simulink model "Sub1"  (R2024a)
settings: Solver=FixedStepDiscrete  StartTime=0.0  StopTime=1  FixedStep=7.5e-05  RelTol=1e-3  EnableMultiTasking=on
undefined symbols (not defined in the file or in its folder): D1, D11, Delta
libraries: spsSeriesRLCBranchLib x41, spsLoadFlowBusLib x29, spsDistributedParametersLineLib x19, spsThreePhaseSeriesRLCLoadLib x15, spsThreePhaseTransformerTwoWindingsLib x13, spsThreePhaseParallelRLCLoadLib x11, spsThreePhaseVIMeasurementLib x11, spsSynchronousMachinepuStandardLib x7, spsExcitationSystemLib x7, spsHydraulicTurbineandGovernorLib x7, spsGenericPowerSystemStabilizerLib x7, spsMultiBandPowerSystemStabilizerLib x7
(part 2 of 5)

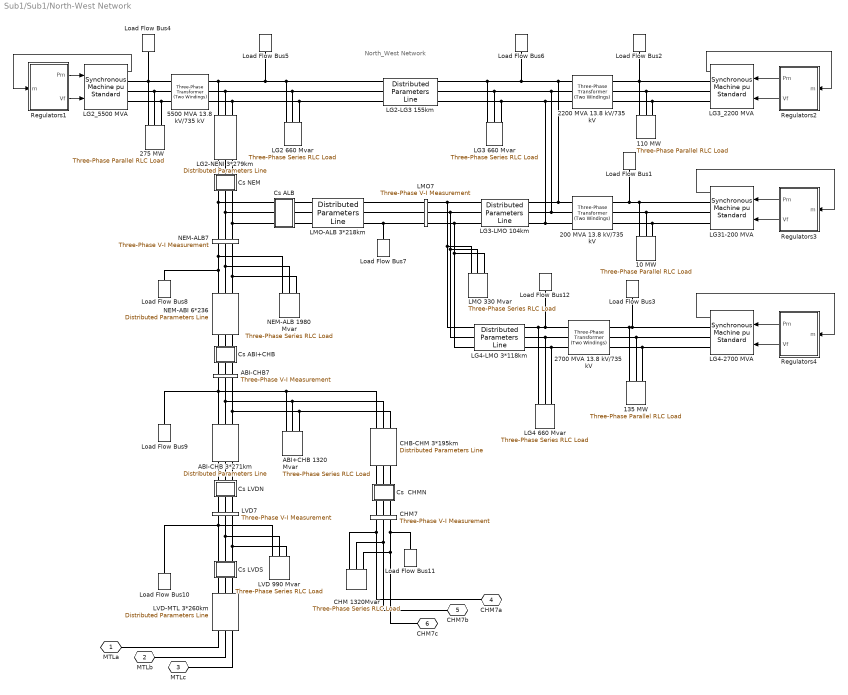
== system Sub1/Sub1/North-West Network ==
  note: North_West Network
  10 MW : spsThreePhaseParallelRLCLoadLib/Three-Phase Parallel RLC Load  LConnTagsString=A|B|C  Configuration=Y (grounded)  NominalVoltage=(13800)*1  Vabc=[1e3 1e3 1e3]  Vabcp=[1e3 1e3 1e3]  NominalFrequency=60  UnbalancedPower=off  ActivePower=10000000  InductivePower=0  CapacitivePower=0  Pabc=[10e3 9e3 11e3]  QLabc=[100 90 110]  QCabc=[100 90 110]  Pabcp=[10e3 9e3 11e3]  QLabcp=[100 90 110]  QCabcp=[100 90 110]  Measurements=None  LoadType=constant PQ
  110 MW : spsThreePhaseParallelRLCLoadLib/Three-Phase Parallel RLC Load  LConnTagsString=A|B|C  Configuration=Y (grounded)  NominalVoltage=(13800)*1  Vabc=[1e3 1e3 1e3]  Vabcp=[1e3 1e3 1e3]  NominalFrequency=60  UnbalancedPower=off  ActivePower=110000000  InductivePower=0  CapacitivePower=0  Pabc=[10e3 9e3 11e3]  QLabc=[100 90 110]  QCabc=[100 90 110]  Pabcp=[10e3 9e3 11e3]  QLabcp=[100 90 110]  QCabcp=[100 90 110]  Measurements=None  LoadType=constant PQ
  135 MW : spsThreePhaseParallelRLCLoadLib/Three-Phase Parallel RLC Load  LConnTagsString=A|B|C  Configuration=Y (grounded)  NominalVoltage=(13800)*1  Vabc=[1e3 1e3 1e3]  Vabcp=[1e3 1e3 1e3]  NominalFrequency=60  UnbalancedPower=off  ActivePower=135000000  InductivePower=0  CapacitivePower=0  Pabc=[10e3 9e3 11e3]  QLabc=[100 90 110]  QCabc=[100 90 110]  Pabcp=[10e3 9e3 11e3]  QLabcp=[100 90 110]  QCabcp=[100 90 110]  Measurements=None  LoadType=constant PQ
  200 MVA 13.8 kV/735 kV : spsThreePhaseTransformerTwoWindingsLib/Three-Phase Transformer (Two Windings)  Winding1Connection=Delta (D1)  Winding2Connection=Yg  CoreType=Three single-phase transformers  SetSaturation=off  Hysteresis=off  DataFile='basic_model'  SetInitialFlux=off  Measurements=None  UNITS=pu  NominalPower=[ 200e6 60 ]  Winding1="[ 13.8e3 0.002  0.0]"  Winding2=[ 735e3 0.002 0.12]  Rm=500  Lm=500  L0=0.5  Saturation="[ 0,0  ;  0.005,1.2  ;  1.0,1.4 ]"  InitialFluxes=[ 0.8 , -0.8 , 0.7 ]  BreakLoop=off  DiscreteSolver=Trapezoidal iterative  DataType=off  TransfoNumber=0
  2200 MVA 13.8 kV/735 kV : spsThreePhaseTransformerTwoWindingsLib/Three-Phase Transformer (Two Windings)  Winding1Connection=Delta (D1)  Winding2Connection=Yg  CoreType=Three single-phase transformers  SetSaturation=off  Hysteresis=off  DataFile='basic_model'  SetInitialFlux=off  Measurements=None  UNITS=pu  NominalPower=[ 2200e6 60 ]  Winding1="[ 13.8e3 0.002  0.0]"  Winding2=[ 735e3 0.002 0.12]  Rm=500  Lm=500  L0=0.5  Saturation="[ 0,0  ;  0.005,1.2  ;  1.0,1.4 ]"  InitialFluxes=[ 0.8 , -0.8 , 0.7 ]  BreakLoop=off  DiscreteSolver=Trapezoidal iterative  DataType=off  TransfoNumber=0
  2700 MVA 13.8 kV/735 kV : spsThreePhaseTransformerTwoWindingsLib/Three-Phase Transformer (Two Windings)  Winding1Connection=Delta (D1)  Winding2Connection=Yg  CoreType=Three single-phase transformers  SetSaturation=off  Hysteresis=off  DataFile='basic_model'  SetInitialFlux=off  Measurements=None  UNITS=pu  NominalPower=[ 2700e6 60 ]  Winding1="[ 13.8e3 0.002  0.0]"  Winding2=[ 735e3 0.002 0.12]  Rm=500  Lm=500  L0=0.5  Saturation="[ 0,0  ;  0.005,1.2  ;  1.0,1.4 ]"  InitialFluxes=[ 0.8 , -0.8 , 0.7 ]  BreakLoop=off  DiscreteSolver=Trapezoidal iterative  DataType=off  TransfoNumber=0
  275 MW : spsThreePhaseParallelRLCLoadLib/Three-Phase Parallel RLC Load  LConnTagsString=A|B|C  Configuration=Y (grounded)  NominalVoltage=(13800)*1  Vabc=[1e3 1e3 1e3]  Vabcp=[1e3 1e3 1e3]  NominalFrequency=60  UnbalancedPower=off  ActivePower=275000000  InductivePower=0  CapacitivePower=0  Pabc=[10e3 9e3 11e3]  QLabc=[100 90 110]  QCabc=[100 90 110]  Pabcp=[10e3 9e3 11e3]  QLabcp=[100 90 110]  QCabcp=[100 90 110]  Measurements=None  LoadType=constant PQ
  5500 MVA 13.8 kV/735 kV : spsThreePhaseTransformerTwoWindingsLib/Three-Phase Transformer (Two Windings)  Winding1Connection=Delta (D1)  Winding2Connection=Yg  CoreType=Three single-phase transformers  SetSaturation=off  Hysteresis=off  DataFile='basic_model'  SetInitialFlux=off  Measurements=None  UNITS=pu  NominalPower=[ 5500e6 60 ]  Winding1="[ 13.8e3 0.002  0.0]"  Winding2=[ 735e3 0.002 0.12]  Rm=500  Lm=500  L0=0.5  Saturation="[ 0,0  ;  0.005,1.2  ;  1.0,1.4 ]"  InitialFluxes=[ 0.8 , -0.8 , 0.7 ]  BreakLoop=off  DiscreteSolver=Trapezoidal iterative  DataType=off  TransfoNumber=0
  ABI+CHB 1320 Mvar : spsThreePhaseSeriesRLCLoadLib/Three-Phase Series RLC Load  LConnTagsString=A|B|C  Configuration=Y (grounded)  NominalVoltage=735e3  Vabc=[1e3 1e3 1e3]  Vabcp=[1e3 1e3 1e3]  NominalFrequency=60  UnbalancedPower=off  ActivePower=4400000  InductivePower=1320e6  CapacitivePower=0  Pabc=[10e3 9e3 11e3]  QLabc=[100 90 110]  QCabc=[100 90 110]  Pabcp=[10e3 9e3 11e3]  QLabcp=[100 90 110]  QCabcp=[100 90 110]  Measurements=None  LoadType=constant Z
  ABI-CHB 3*271km : spsDistributedParametersLineLib/Distributed Parameters Line  Phases=3  Length=271  Frequency=60  Resistance="[0.01273  0.3864]/3"  Inductance="[0.9337e-3  4.1264e-3]/3"  Capacitance=[12.74e-9 7.751e-9]*3  x1=[-0.001575 2.7348412269526e-08 -34814.2579741144 -747194.944177871;-0.0015 2.74950573148694e-08 -13676.7298714156 -747880.497252537;-0.001425 2.76197232320838e-08 7471.73119988141 -747968.206100654;-0.00135 2.77223103651424e-08 28614.2194835787 -747458.000609112;-0.001275 2.78027367074606e-08 49733.8339980329 -746350.288628374;-0.0012 2.78609379674511e-08 70813.6920465424 -744645.955646449;-0.001125 2.7896867619917e-08 91836.9427131156 -742346.364081045;-0.00105 2.7910496943244e-08 112786.780332836 -739453.352190476;-0.000975 2.79018150423594e-08 133646.457926055 -735969.23260418;-0.0009 2.78708288574421e-08 154399.300585666 -731896.790474048;-0.000825 2.78175631583741e-08 175028.718806778 -727239.281248007;-0.00075 2.77420605249403e-08 195518.221748105 -722000.428067671;-0.000675 2.76443813127906e-08 215851.430414496 -716184.418792115;-0.0006 2.75246036051927e-08 236012.09075005 -709795.902650165;-0.000525 2.73828231506133e-08 255984.086631366 -702839.986523878;-0.00045 2.72191532861786e-08 275751.452750516 -695322.230866176;-0.000375 2.7033724847074e-08 295298.387377476 -687248.645255907;-0.0003 2.68266860619564e-08 314609.264991783 -678625.683593877;-0.000225 2.6598202434463e-08 333668.64877334 -669460.238943703;-0.00015 2.63484566109096e-08 352461.302942368 -659759.638021603;-7.5e-05 2.60776482342864e-08 370972.204938663 -649531.635339529]  x2=[-0.001575 6.20449125576539e-08 -284619.341076147 -691578.758256562;-0.0015 6.22834048516216e-08 -264954.25531134 -699348.683850865;-0.001425 6.2472108744719e-08 -245077.369168772 -706559.560807692;-0.00135 6.26108733899411e-08 -225004.5719271 -713205.624862332;-0.001275 6.26995878609538e-08 -204751.909473316 -719281.56325287;-0.0012 6.27381812407664e-08 -184335.571475907 -724782.518967121;-0.001125 6.27266226784214e-08 -163771.87844309 -729704.094625253;-0.00105 6.26649214136568e-08 -143077.268676438 -734042.355994989;-0.000975 6.25531267695196e-08 -122268.285130363 -737793.835136568;-0.0009 6.23913281129378e-08 -101361.562187922 -740955.533174962;-0.000825 6.21796547832818e-08 -80373.8123635515 -743524.922697137;-0.00075 6.19182759889726e-08 -59321.8129433384 -745499.949772419;-0.000675 6.16074006722193e-08 -38222.3925735125 -746879.035594386;-0.0006 6.12472773419935e-08 -17092.4178078855 -747661.077742931;-0.000525 6.08381938753752e-08 4051.22037501424 -747845.451065526;-0.00045 6.03804772874285e-08 25191.620074332 -747432.008176959;-0.000375 5.98744934697906e-08 46311.8819780071 -746421.079577148;-0.0003 5.93206468981833e-08 67395.1228718245 -744813.473386949;-0.000225 5.8719380309082e-08 88424.489135598 -742610.474702152;-0.00015 5.80711743457983e-08 109383.170215697 -739813.8445662;-7.5e-05 5.73765471742613e-08 130254.412063144 -736425.818562433]  x3=[-0.001575 1.23942804838449e-10 -354.964030660947 -109.750554352367;-0.0015 1.32024870831634e-10 -351.719210477296 -119.741131836523;-0.001425 1.40001398163125e-10 -348.193231338274 -129.63599009199;-0.00135 1.47866010519017e-10 -344.388911857655 -139.427219320474;-0.001275 1.55612421048526e-10 -340.309293150224 -149.106992563141;-0.0012 1.63234437389599e-10 -335.957636400756 -158.667571957367;-0.001125 1.70725966618993e-10 -331.337420257073 -168.101314922266;-0.00105 1.78081020122867e-10 -326.452338049269 -177.400680268052;-0.000975 1.85293718383986e-10 -321.306294837316 -186.558234224353;-0.0009 1.92358295681718e-10 -315.903404289422 -195.566656382652;-0.000825 1.99269104701062e-10 -310.247985393623 -204.418745548109;-0.00075 2.06020621047027e-10 -304.344559005254 -213.107425496086;-0.000675 2.12607447660749e-10 -298.197844233044 -221.625750628775;-0.0006 2.19024319133814e-10 -291.812754666734 -229.966911527399;-0.000525 2.25266105917348e-10 -285.194394449229 -238.12424039556;-0.00045 2.31327818422499e-10 -278.348054196421 -246.091216389371;-0.000375 2.37204611009036e-10 -271.279206767956 -253.861470830122;-0.0003 2.42891785858886e-10 -263.993502892313 -261.428792295303;-0.000225 2.48384796731489e-10 -256.496766649693 -268.787131583918;-0.00015 2.53679252597999e-10 -248.794990816346 -275.930606552125;-7.5e-05 2.58770921151406e-10 -240.894332074031 -282.853506815335]  x4=[-0.001575 1.87538445523221e-10 -5971.27343085295 -15054.8004559032;-0.0015 1.8367258103474e-10 -5543.27939856625 -15217.5948036276;-0.001425 1.79659891495264e-10 -5110.85415354334 -15368.224438903;-0.00135 1.75503584587415e-10 -4674.34336990879 -15506.5689507036;-0.001275 1.71206982799342e-10 -4234.09598770418 -15632.5177485435;-0.0012 1.66773520768774e-10 -3790.46393395085 -15745.9701508808;-0.001125 1.62206742537423e-10 -3343.80184132475 -15846.8354656009;-0.00105 1.57510298717935e-10 -2894.46676466859 -15935.0330625145;-0.000975 1.5268794357564e-10 -2442.81789556757 -16010.492437812;-0.0009 1.47743532027454e-10 -1989.21627521721 -16073.1532704236;-0.000825 1.42681016560317e-10 -1534.02450581247 -16122.9654702383;-0.00075 1.37504444071635e-10 -1077.60646068914 -16159.8892181457;-0.000675 1.32217952634251e-10 -620.326993449071 -16183.8949978667;-0.0006 1.26825768188533e-10 -162.55164630176 -16194.9636195483;-0.000525 1.21332201164225e-10 295.353642144482 -16193.0862351037;-0.00045 1.15741643034751e-10 753.022829408257 -16178.2643452853;-0.000375 1.10058562806741e-10 1210.09006174384 -16150.509798485;-0.0003 1.04287503447577e-10 1666.18996659906 -16109.8447812629;-0.000225 9.84330782538081e-11 2120.95794468854 -16056.3018006115;-0.00015 9.24999671633602e-11 2574.03046144879 -15989.9236579704;-7.5e-05 8.64929130144588e-11 3025.04533764214 -15910.7634150111]  x5=0.00153261764655846  V1=ones(3,3)  V2=ones(3,3)  I1=ones(3,3)  I2=ones(3,3)  nHarmo=1  Measurements=None  Decoupling=on  VsMag0=[610743.955114558 610743.501374985 610743.958217937]  VrMag0=[610622.36047804 610622.247686735 610622.21400359]  VsAngle0=[1.35232982186252 -118.647645266066 121.352379141748]  VrAngle0=[-18.3496130787498 -138.349622838584 101.650391206839]  IsMag0=[305.299965908709 305.301188713838 305.286778308251]  IrMag0=[13308.3117169382 13308.3164139121 13308.3246262135]  IsAngle0=[-68.7963830004883 171.200626739938 51.2019231188552]  IrAngle0=[-17.6151010152126 -137.615048514485 102.384907722662]
      settings: AttributesFormatString=\n  LibrarySourceBlock=sps_lib/Power Grid Elements/Distributed Parameters Line
  ABI-CHB7 : spsThreePhaseVIMeasurementLib/Three-Phase V-I Measurement  VoltageMeasurement=no  SetLabelV=on  LabelV=Vabc_ABI7  Vpu=on  VpuLL=off  CurrentMeasurement=no  SetLabelI=off  LabelI=A1  Ipu=off  Pbase=100e6  Vbase=500e3  OutputType=Magnitude  PhasorSimulation=off  PSBequivalent=0
  CHB-CHM 3*195km : spsDistributedParametersLineLib/Distributed Parameters Line  Phases=3  Length=195  Frequency=60  Resistance="[0.01273  0.3864]/3"  Inductance="[0.9337e-3  4.1264e-3]/3"  Capacitance=[12.74e-9 7.751e-9]*3  x1=[-0.001125 2.7896867619917e-08 0 0;-0.00105 2.7910496943244e-08 0 0;-0.000975 2.79018150423594e-08 0 0;-0.0009 2.78708288574421e-08 0 0;-0.000825 2.78175631583741e-08 0 0;-0.00075 2.77420605249403e-08 0 0;-0.000675 2.76443813127906e-08 215851.430414496 -716184.418792115;-0.0006 2.75246036051927e-08 236012.09075005 -709795.902650165;-0.000525 2.73828231506133e-08 255984.086631366 -702839.986523878;-0.00045 2.72191532861786e-08 275751.452750516 -695322.230866176;-0.000375 2.7033724847074e-08 295298.387377476 -687248.645255907;-0.0003 2.68266860619564e-08 314609.264991783 -678625.683593877;-0.000225 2.6598202434463e-08 333668.64877334 -669460.238943703;-0.00015 2.63484566109096e-08 352461.302942368 -659759.638021603;-7.5e-05 2.60776482342864e-08 370972.204938663 -649531.635339529]  x2=[-0.001125 1.96074578395808e-08 0 0;-0.00105 1.95835879445984e-08 0 0;-0.000975 1.95440632290521e-08 0 0;-0.0009 1.94889152883947e-08 0 0;-0.000825 1.94181882070461e-08 0 0;-0.00075 1.93319385231531e-08 0 0;-0.000675 1.92302351833932e-08 127559.107191232 -726636.134488282;-0.0006 1.91131594878602e-08 148050.539525855 -722739.535822949;-0.000525 1.89808050250737e-08 168423.622524431 -718265.190230966;-0.00045 1.88332775971663e-08 188662.070256128 -713216.674435737;-0.000375 1.86706951353065e-08 208749.704415489 -707598.024143546;-0.0003 1.84931876054267e-08 228670.467255118 -701413.730817467;-0.000225 1.83008969043304e-08 248408.434421998 -694668.738086963;-0.00015 1.80939767462619e-08 267947.827687178 -687368.43779602;-7.5e-05 1.78725925400296e-08 287273.027558644 -679518.665692993]  x3=[-0.001125 1.01533523421544e-10 0 0;-0.00105 9.99122586246718e-11 0 0;-0.000975 9.82111254969635e-11 0 0;-0.0009 9.64314838982135e-11 0 0;-0.000825 9.45747564466865e-11 0 0;-0.00075 9.26424273818983e-11 0 0;-0.000675 9.06360413781377e-11 771.180648774585 -4323.83757003266;-0.0006 8.85572023096773e-11 893.1105985654 -4300.30718909003;-0.000525 8.64075719686612e-11 1014.32660940877 -4273.33920837735;-0.00045 8.41888687366936e-11 1134.7317830803 -4242.95518568578;-0.000375 8.19028662111907e-11 1254.22986952641 -4209.17940953816;-0.0003 7.95513917875944e-11 1372.72534380519 -4172.03887977315;-0.000225 7.71363251985803e-11 1490.12348244752 -4131.563285962;-0.00015 7.46595970114278e-11 1606.33043917765 -4087.78498367508;-7.5e-05 7.21231870847545e-11 1721.25331993237 -4040.73896861743]  x4=[-0.001125 7.61596569036021e-11 0 0;-0.00105 7.88963891504129e-11 0 0;-0.000975 8.1570052830892e-11 0 0;-0.0009 8.41785106592017e-11 0 0;-0.000825 8.67196774740649e-11 0 0;-0.00075 8.91915219056109e-11 0 0;-0.000675 9.15920679992215e-11 979.60695261617 -12037.6056406799;-0.0006 9.39193967950793e-11 1319.52443201652 -12005.1005057388;-0.000525 9.6171647862154e-11 1658.38710377532 -11962.9986771376;-0.00045 9.83470207854032e-11 1995.92408625753 -11911.333810434;-0.000375 1.00443776604997e-10 2331.86555756385 -11850.1472057317;-0.0003 1.02460239206413e-10 2665.94297122219 -11779.4877746666;-0.000225 1.04394796660302e-10 2997.88927085963 -11699.4120013066;-0.00015 1.06245902511035e-10 3327.4391036832 -11609.9838969998;-7.5e-05 1.08012077012918e-10 3654.3290325988 -11511.2749492044]  x5=0.0011028060556417  V1=ones(3,3)  V2=ones(3,3)  I1=ones(3,3)  I2=ones(3,3)  nHarmo=1  Measurements=None  Decoupling=on  VsMag0=[610743.955114558 610743.501374985 610743.958217937]  VrMag0=[602368.350238942 602368.356498648 602368.322152075]  VsAngle0=[1.35232982186252 -118.647645266066 121.352379141748]  VrAngle0=[-5.46332293594696 -125.463326364553 114.536674834112]  IsMag0=[3602.61669203512 3602.60152789018 3602.59275066703]  IrMag0=[9906.44607872302 9906.45414351731 9906.46948058143]  IsAngle0=[-5.30716137480681 -125.307461802367 114.69289727209]  IrAngle0=[-10.7676510977489 -130.767521740262 109.232373186016]
      settings: AttributesFormatString=\n  LibrarySourceBlock=sps_lib/Power Grid Elements/Distributed Parameters Line
  CHM 1320Mvar : spsThreePhaseSeriesRLCLoadLib/Three-Phase Series RLC Load  LConnTagsString=A|B|C  Configuration=Y (grounded)  NominalVoltage=735e3  Vabc=[1e3 1e3 1e3]  Vabcp=[1e3 1e3 1e3]  NominalFrequency=60  UnbalancedPower=off  ActivePower=4400000  InductivePower=1320e6  CapacitivePower=0  Pabc=[10e3 9e3 11e3]  QLabc=[100 90 110]  QCabc=[100 90 110]  Pabcp=[10e3 9e3 11e3]  QLabcp=[100 90 110]  QCabcp=[100 90 110]  Measurements=None  LoadType=constant Z
  CHM7 : spsThreePhaseVIMeasurementLib/Three-Phase V-I Measurement  VoltageMeasurement=no  SetLabelV=on  LabelV=Vabc_CHM7  Vpu=on  VpuLL=off  CurrentMeasurement=no  SetLabelI=off  LabelI=A1  Ipu=off  Pbase=100e6  Vbase=735e3  OutputType=Magnitude  PhasorSimulation=off  PSBequivalent=0
  "Cs  CHMN " : Subsystem  mask{Xc=25/3}
      mask prompts: Xc "Condensator Reactance at  60Hz  (ohm):"
      mask help: Series Compensation
      mask init:
      | Cs=1/Xc/(2*pi*60);
      mask Display: disp('Cs')
  "Cs ABI+CHB " : Subsystem  mask{Xc=25/6}
      mask prompts: Xc "Condensator Reactance at  60Hz  (ohm):"
      mask help: Series Compensation
      mask init:
      | Cs=1/Xc/(2*pi*60);
      mask Display: disp('Cs')
  Cs ALB : Subsystem  mask{Xc=16/3}
      mask prompts: Xc "Reactance @ 60Hz du condensateur (ohm):"
      mask init:
      | Cs=1/Xc/(2*pi*60);
      mask Display: disp('Cs')
  "Cs LVDN " : Subsystem  mask{Xc=34/3}
      mask prompts: Xc "Condensator Reactance at  60Hz  (ohm):"
      mask help: Series Compensation
      mask init:
      | Cs=1/Xc/(2*pi*60);
      mask Display: disp('Cs')
  "Cs LVDS " : Subsystem  mask{Xc=34/3}
      mask prompts: Xc "Condensator Reactance at  60Hz  (ohm):"
      mask help: Series Compensation
      mask init:
      | Cs=1/Xc/(2*pi*60);
      mask Display: disp('Cs')
  "Cs NEM " : Subsystem  mask{Xc=16/3}
      mask prompts: Xc "Condensator Reactance at  60Hz  (ohm):"
      mask help: Series Compensation
      mask init:
      | Cs=1/Xc/(2*pi*60);
      mask Display: disp('Cs')
  LG2 660 Mvar : spsThreePhaseSeriesRLCLoadLib/Three-Phase Series RLC Load  LConnTagsString=A|B|C  Configuration=Y (grounded)  NominalVoltage=735e3  Vabc=[1e3 1e3 1e3]  Vabcp=[1e3 1e3 1e3]  NominalFrequency=60  UnbalancedPower=off  ActivePower=2200000  InductivePower=660e6  CapacitivePower=0  Pabc=[10e3 9e3 11e3]  QLabc=[100 90 110]  QCabc=[100 90 110]  Pabcp=[10e3 9e3 11e3]  QLabcp=[100 90 110]  QCabcp=[100 90 110]  Measurements=None  LoadType=constant Z
  LG2-LG3 155km : spsDistributedParametersLineLib/Distributed Parameters Line  Phases=3  Length=155  Frequency=60  Resistance="[0.01273  0.3864]"  Inductance="[0.9337e-3  4.1264e-3]"  Capacitance=[12.74e-9 7.751e-9]  x1=[-0.0009 5.14991398324284e-10 425726.576739804 -584301.004479446;-0.000825 5.6006015518295e-10 442074.91123423 -572031.872777778;-0.00075 6.04681208522771e-10 458069.857808588 -559305.467549392;-0.000675 6.48818888956431e-10 473698.630347318 -546131.962087907;-0.0006 6.92437913497522e-10 488948.73544878 -532521.887092029;-0.000525 7.35503413765218e-10 503807.982412291 -518486.122247467;-0.00045 7.77980963857529e-10 518264.492983182 -504035.887529885;-0.000375 8.19836607870841e-10 532306.710848095 -489182.734235818;-0.0003 8.61036887043742e-10 545923.410872923 -473938.535748751;-0.000225 9.01548866503446e-10 559103.708076006 -458315.478047709;-0.00015 9.41340161593427e-10 571837.066329427 -442326.049965977;-7.5e-05 9.80378963761218e-10 584113.306781425 -425983.033207718]  x2=[-0.0009 -3.80996883150677e-10 428602.512418851 -576982.581433426;-0.000825 -4.1954707898371e-10 444742.801992321 -564635.073573809;-0.00075 -4.57761895301089e-10 460527.570974672 -551836.205075583;-0.000675 -4.95610783763356e-10 475944.201263094 -538596.207158396;-0.0006 -5.33063488548182e-10 490980.369039216 -524925.663674006;-0.000525 -5.70090070536408e-10 505624.05462058 -510835.502645706;-0.00045 -6.06660931244917e-10 519863.552068988 -496336.987532636;-0.000375 -6.42746836487213e-10 533687.478548051 -481441.708225944;-0.0003 -6.78318939742777e-10 547084.783422455 -466161.571784001;-0.000225 -7.13348805216538e-10 560044.757091669 -450508.792914085;-0.00015 -7.47808430570012e-10 572557.039551036 -434495.884208129;-7.5e-05 -7.81670269305942e-10 584611.628673402 -418135.646140348]  x3=[-0.0009 1.08886136484288e-11 1482.81916403291 -2352.94053779496;-0.000825 1.07442931700891e-11 1548.74539245887 -2310.07973089038;-0.00075 1.05913838681825e-11 1613.4335775147 -2265.37228159434;-0.000675 1.04300079760653e-11 1676.83200845502 -2218.85392835774;-0.0006 1.02602944951565e-11 1738.89000554418 -2170.56185724042;-0.000525 1.0082379091816e-11 1799.55796056881 -2120.53467218514;-0.00045 9.89640398889509e-12 1858.78737649393 -2068.81236415817;-0.000375 9.70251785204551e-12 1916.53090623067 -2015.43627918119;-0.0003 9.50087567087852e-12 1972.74239048488 -1960.44908527984;-0.000225 9.2916386350685e-12 2027.37689465611 -1903.8947383756;-0.00015 9.07497400550044e-12 2080.39074475766 -1845.81844714806;-7.5e-05 8.85105498056414e-12 2131.74156232889 -1786.26663689584]  x4=[-0.0009 -1.26559708510045e-11 1223.55408119253 -2231.14873574737;-0.000825 -1.24991373349499e-11 1286.14070278666 -2195.66620561399;-0.00075 -1.2332312199753e-11 1347.6992031816 -2158.42849351067;-0.000675 -1.21556288028742e-11 1408.18037345401 -2119.4653666947;-0.0006 -1.19692283823178e-11 1467.53586588176 -2078.8079716935;-0.000525 -1.17732599437279e-11 1525.71823259237 -2036.48880940655;-0.00045 -1.1567880141276e-11 1582.68096349213 -1992.54170912469;-0.000375 -1.13532531524335e-11 1638.37852344549 -1947.00180148747;-0.0003 -1.11295505467317e-11 1692.76638867525 -1899.90549040026;-0.000225 -1.08969511486106e-11 1745.8010823541 -1851.29042393356;-0.00015 -1.06556408944702e-11 1797.44020935936 -1801.19546422766;-7.5e-05 -1.04058126840356e-11 1847.64249016302 -1749.66065642687]  x5=0.000876589428843401  V1=ones(3,3)  V2=ones(3,3)  I1=ones(3,3)  I2=ones(3,3)  nHarmo=1  Measurements=None  Decoupling=on  VsMag0=[590283.056617457 590282.243891804 590283.870916768]  VrMag0=[586861.315379361 586860.56906448 586862.120536081]  VsAngle0=[25.5173905041513 -94.4824726828201 145.517527228803]  VrAngle0=[26.0462334057304 -93.9536337576226 146.046362925454]  IsMag0=[2279.13376434155 2279.13000762751 2279.13554694022]  IrMag0=[2085.26033535343 2085.25824212114 2085.26456016713]  IsAngle0=[21.6590596698427 -98.3408340586465 141.659194593867]  IrAngle0=[18.1802070278353 -101.819625724336 138.180340460903]
      settings: AttributesFormatString=\n  LibrarySourceBlock=sps_lib/Power Grid Elements/Distributed Parameters Line
  LG2-NENI 3*279km : spsDistributedParametersLineLib/Distributed Parameters Line  Phases=3  Length=279  Frequency=60  Resistance="[0.01273  0.3864]/3"  Inductance="[0.9337e-3  4.1264e-3]/3"  Capacitance=[12.74e-9 7.751e-9]*3  x1=[-0.00165 4.77458143840719e-11 245808.020606762 -679875.080306638;-0.001575 9.52654974816539e-11 264930.184927427 -672654.157661194;-0.0015 1.4270902679816e-10 283840.56811183 -664895.52557407;-0.001425 1.90038476702166e-10 302524.05348899 -656605.386177045;-0.00135 2.37216012755581e-10 320965.705766564 -647790.366480709;-0.001275 2.84203921957927e-10 339150.782969888 -638457.513076933;-0.0012 3.30964642893525e-10 357064.748226487 -628614.286505931;-0.001125 3.77460795757523e-10 374693.281386628 -618268.555292418;-0.00105 4.23655212236737e-10 392022.290470628 -607428.589655629;-0.000975 4.6951096522143e-10 409037.922933767 -596103.054898239;-0.0009 5.14991398324284e-10 425726.576739804 -584301.004479446;-0.000825 5.6006015518295e-10 442074.91123423 -572031.872777778;-0.00075 6.04681208522771e-10 458069.857808588 -559305.467549392;-0.000675 6.48818888956431e-10 473698.630347318 -546131.962087907;-0.0006 6.92437913497522e-10 488948.73544878 -532521.887092029;-0.000525 7.35503413765218e-10 503807.982412291 -518486.122247467;-0.00045 7.77980963857529e-10 518264.492983182 -504035.887529885;-0.000375 8.19836607870841e-10 532306.710848095 -489182.734235818;-0.0003 8.61036887043742e-10 545923.410872923 -473938.535748751;-0.000225 9.01548866503446e-10 559103.708076006 -458315.478047709;-0.00015 9.41340161593427e-10 571837.066329427 -442326.049965977;-7.5e-05 9.80378963761218e-10 584113.306781425 -425983.033207718]  x2=[-0.00165 1.65880252234434e-08 25617.0786733438 -737924.872188863;-0.001575 1.66898350173596e-08 46468.3767746556 -736905.697758344;-0.0015 1.67783032125259e-08 67282.5287665638 -735297.452188073;-0.001425 1.68533590888207e-08 88042.8961344332 -733101.421084951;-0.00135 1.6914942647725e-08 108732.883358234 -730319.359922642;-0.001275 1.6963004660284e-08 129335.951178748 -726953.492638272;-0.0012 1.69975067064603e-08 149835.629818795 -723006.509854648;-0.001125 1.70184212058459e-08 170215.532148928 -718481.566729416;-0.00105 1.70257314397103e-08 190459.366787045 -713382.280432878;-0.000975 1.70194315643641e-08 210550.951121479 -707712.727256476;-0.0009 1.69995266158314e-08 230474.224247124 -701477.439354274;-0.000825 1.69660325058235e-08 250213.25980428 -694681.401120017;-0.00075 1.69189760090194e-08 269752.278709939 -687330.045202686;-0.000675 1.68583947416628e-08 289075.661771346 -679429.248163722;-0.0006 1.67843371314917e-08 308167.962171739 -670985.325779392;-0.000525 1.66968623790267e-08 327013.9178183 -662005.027992054;-0.00045 1.65960404102465e-08 345598.463542438 -652495.533514356;-0.000375 1.64819518206902e-08 363906.743142653 -642464.444090683;-0.0003 1.63546878110308e-08 381924.12126036 -631919.77842044;-0.000225 1.62143501141704e-08 399636.195079167 -620869.965748024;-0.00015 1.60610509139166e-08 417028.805838266 -609323.839124618;-7.5e-05 1.58949127553045e-08 434088.050150733 -597290.628347183]  x3=[-0.00165 7.88000012065198e-12 -714.300687613336 -1196.52974167661;-0.001575 1.11572333167731e-11 -680.188293410607 -1216.24398928443;-0.0015 1.44255475912921e-11 -645.532167093356 -1234.98599005637;-0.001425 1.7682330303785e-11 -610.360012238703 -1252.74076192378;-0.00135 2.09249780319818e-11 -574.699944929088 -1269.49411199368;-0.001275 2.41508986529026e-11 -538.580471276701 -1285.23264789437;-0.0012 2.73575134149615e-11 -502.030464636132 -1299.94378848105;-0.001125 3.05422589993805e-11 -465.079142523458 -1313.61577389303;-0.00105 3.37025895692676e-11 -427.756043260199 -1326.23767495435;-0.000975 3.68359788047199e-11 -390.091002360845 -1337.79940191043;-0.0009 3.99399219223251e-11 -352.114128682797 -1348.29171249364;-0.000825 4.30119376774469e-11 -313.855780357806 -1357.70621931143;-0.00075 4.60495703476941e-11 -275.346540524152 -1366.03539655111;-0.000675 4.90503916959874e-11 -236.617192878946 -1373.27258599583;-0.0006 5.2012002911655e-11 -197.698697070117 -1379.41200234708;-0.000525 5.49320365280054e-11 -158.622163947742 -1384.44873784937;-0.00045 5.78081583148437e-11 -119.418830694507 -1388.37876621339;-0.000375 6.06380691444196e-11 -80.1200358551849 -1391.19894583461;-0.0003 6.3419506829315e-11 -40.7571942850775 -1392.90702230459;-0.000225 6.6150247930802e-11 -1.36177203746462 -1393.50163021313;-0.00015 6.88281095362259e-11 38.0347387898792 -1392.98229423977;-7.5e-05 7.14509510039919e-11 77.4008452289855 -1391.34942953374]  x4=[-0.00165 4.32486862614941e-11 829.758142041681 -14907.5065102212;-0.001575 4.09933442212519e-11 1250.86903709497 -14878.090885747;-0.0015 3.87052327288585e-11 1670.98000657895 -14836.7819430612;-0.001425 3.63861808656315e-11 2089.75522021252 -14783.6127039005;-0.00135 3.40380424461478e-11 2506.85991549738 -14718.6256709412;-0.001275 3.16626945363322e-11 2921.96066532203 -14641.872793823;-0.0012 2.92620359529597e-11 3334.72564449832 -14553.4154276216;-0.001125 2.68379857457706e-11 3744.82489501741 -14453.3242838022;-0.00105 2.43924816634112e-11 4151.93058981317 -14341.6793736935;-0.000975 2.19274786044276e-11 4555.7172948221 -14218.5699445285;-0.0009 1.94449470545493e-11 4955.86222913036 -14084.0944081013;-0.000825 1.69468715115132e-11 5352.04552299989 -13938.3602620981;-0.00075 1.44352488986867e-11 5743.95047356738 -13781.4840041655;-0.000675 1.19120869687573e-11 6131.26379801168 -13613.5910387837;-0.0006 9.37940269876608e-12 6513.67588398734 -13434.8155770204;-0.000525 6.83922067776716e-12 6890.88103712392 -13245.3005292445;-0.00045 4.29357148840201e-12 7262.57772539344 -13045.1973908853;-0.000375 1.74449008368288e-12 7628.46882015044 -12834.6661213301;-0.0003 -8.05985839717548e-13 7988.2618336521 -12613.8750160545;-0.000225 -3.3558174703697e-12 8341.66915286845 -12383.0005720898;-0.00015 -5.90296651188178e-12 8688.40826939581 -12142.227346934;-7.5e-05 -8.44539681228267e-12 9028.20200528972 -11891.7478110194]  x5=0.00157786097191812  V1=ones(3,3)  V2=ones(3,3)  I1=ones(3,3)  I2=ones(3,3)  nHarmo=1  Measurements=None  Decoupling=on  VsMag0=[590283.056617457 590282.243891804 590283.870916768]  VrMag0=[602875.980203818 602875.441014933 602876.102194564]  VsAngle0=[25.5173905041513 -94.4824726828201 145.517527228803]  VrAngle0=[7.62822080532787 -112.371736222205 127.628286669388]  IsMag0=[1145.30812027455 1145.28643709992 1145.27794996152]  IrMag0=[12270.9673380102 12270.9820903542 12270.998354886]  IsAngle0=[-25.1951184881794 -145.196235040903 94.805262672481]  IrAngle0=[8.82574494857866 -111.174127591585 128.825749025247]
      settings: AttributesFormatString=\n  LibrarySourceBlock=sps_lib/Power Grid Elements/Distributed Parameters Line
  LG2_5500 MVA : spsSynchronousMachinepuStandardLib/Synchronous Machine pu Standard  PresetModel=No  MechanicalLoad=Mechanical power Pm  ShowDetailedParameters=on  RotorType=Salient-pole  Units=per unit standard parameters  MeasurementBus=off  NominalParameters="[5500E6  13800   60 ]"  Reactances1=[ 31 32 33 34 35 36 37 ]  Reactances2=[ 1.305, 0.296, 0.252, 0.474, 0.243, 0.18 ]  dAxisTimeConstants=Short-circuit  qAxisTimeConstants=Open-circuit  TimeConstants1=[]  TimeConstants2=[]  TimeConstants3=[]  TimeConstants4=[]  TimeConstants5=[ 1.01, 0.053, 0.1 ]  TimeConstants6=[]  TimeConstants7=[]  TimeConstants8=[]  StatorResistance=2.8544e-3  Mechanical="[ 4.1  0  32]"  PolePairs=32  InitialConditions=[0 -65.2434 0.985682 0.985682 0.985682 -1.22427 -121.224 118.776 1.47412]  SetSaturation=off  Saturation=[0.6404,0.7127,0.8441,0.9214,0.9956,1.082,1.19,1.316,1.457;0.7,0.7698,0.8872,0.9466,0.9969,1.046,1.1,1.151,1.201]  LoadFlowParameters=[2 4000000000 0 0 0]  TsPowergui=0  TsBlock=-1  IterativeModel=Trapezoidal non iterative  IterativeDiscreteModel=Trapezoidal non iterative  BusType=swing  Pref=0  Qref=0  Qmin=-Inf  Qmax=Inf  PLF=0  QLF=0
  LG3 660 Mvar : spsThreePhaseSeriesRLCLoadLib/Three-Phase Series RLC Load  LConnTagsString=A|B|C  Configuration=Y (grounded)  NominalVoltage=735e3  Vabc=[1e3 1e3 1e3]  Vabcp=[1e3 1e3 1e3]  NominalFrequency=60  UnbalancedPower=off  ActivePower=2200000  InductivePower=660e6  CapacitivePower=0  Pabc=[10e3 9e3 11e3]  QLabc=[100 90 110]  QCabc=[100 90 110]  Pabcp=[10e3 9e3 11e3]  QLabcp=[100 90 110]  QCabcp=[100 90 110]  Measurements=None  LoadType=constant Z
  LG3-LMO 104km : spsDistributedParametersLineLib/Distributed Parameters Line  Phases=3  Length=104  Frequency=60  Resistance="[0.01273  0.3864]"  Inductance="[0.9337e-3  4.1264e-3]"  Capacitance=[12.74e-9 7.751e-9]  x1=[-0.0006 -5.33063488548182e-10 0 0;-0.000525 -5.70090070536408e-10 0 0;-0.00045 -6.06660931244917e-10 0 0;-0.000375 -6.42746836487213e-10 533687.478548051 -481441.708225944;-0.0003 -6.78318939742777e-10 547084.783422455 -466161.571784001;-0.000225 -7.13348805216538e-10 560044.757091669 -450508.792914085;-0.00015 -7.47808430570012e-10 572557.039551036 -434495.884208129;-7.5e-05 -7.81670269305942e-10 584611.628673402 -418135.646140348]  x2=[-0.0006 4.52757114468228e-09 0 0;-0.000525 4.47585472485853e-09 0 0;-0.00045 4.42056037525061e-09 0 0;-0.000375 4.36173229731554e-09 480200.396912793 -552194.743514625;-0.0003 4.29941751731875e-09 495619.314773631 -538398.460516251;-0.000225 4.23366584874191e-09 510642.04213747 -524171.790026312;-0.00015 4.16452985246284e-09 525256.570065909 -509526.104627524;-7.5e-05 4.09206479473916e-09 539451.215928932 -494473.111856707]  x3=[-0.0006 1.00495274917935e-11 0 0;-0.000525 1.08359946018696e-11 0 0;-0.00045 1.16137995836573e-11 0 0;-0.000375 1.23823206717549e-11 -139.986222681574 -514.51577923574;-0.0003 1.31409435221634e-11 -125.384058316502 -518.267255559262;-0.000225 1.38890617033834e-11 -110.681663853653 -521.604436968444;-0.00015 1.46260771811875e-11 -95.8907921622048 -524.52465577153;-7.5e-05 1.53514007966794e-11 -81.0232668386807 -527.025577590288]  x4=[-0.0006 -3.19987947216074e-12 0 0;-0.000525 -3.97660474306703e-12 0 0;-0.00045 -4.7501511769858e-12 0 0;-0.000375 -5.51990041273344e-12 3613.50960647477 -3542.58660366421;-0.0003 -6.28523712454845e-12 3712.21557844744 -3439.014704798;-0.000225 -7.04554951397345e-12 3807.9540620855 -3332.69371019546;-0.00015 -7.8002297989175e-12 3900.64852550998 -3223.70861123291;-7.5e-05 -8.54867469950781e-12 3990.22487018509 -3112.14652893094]  x5=0.000588163229675572  V1=ones(3,3)  V2=ones(3,3)  I1=ones(3,3)  I2=ones(3,3)  nHarmo=1  Measurements=None  Decoupling=on  VsMag0=[586861.315379361 586860.56906448 586862.120536081]  VrMag0=[597501.49549937 597500.918482429 597501.873521745]  VsAngle0=[26.0462334057304 -93.9536337576226 146.046362925454]  VrAngle0=[19.1109154470794 -100.889010750024 139.111000266937]  IsMag0=[436.45107990204 436.445924432083 436.434679858475]  IrMag0=[4141.87607401795 4141.88820061754 4141.89211373189]  IsAngle0=[-37.1184575596386 -157.120552820034 82.8810809575759]  IrAngle0=[23.6678939918001 -96.3319466522339 143.667828394019]
      settings: AttributesFormatString=\n  LibrarySourceBlock=sps_lib/Power Grid Elements/Distributed Parameters Line
  LG31-200 MVA : spsSynchronousMachinepuStandardLib/Synchronous Machine pu Standard  PresetModel=No  MechanicalLoad=Mechanical power Pm  ShowDetailedParameters=on  RotorType=Salient-pole  Units=per unit standard parameters  MeasurementBus=off  NominalParameters="[200E6  13800   60 ]"  Reactances1=[ 31 32 33 34 35 36 37 ]  Reactances2=[ 1.305, 0.296, 0.252, 0.474, 0.243, 0.18 ]  dAxisTimeConstants=Short-circuit  qAxisTimeConstants=Open-circuit  TimeConstants1=[]  TimeConstants2=[]  TimeConstants3=[]  TimeConstants4=[]  TimeConstants5=[ 1.01, 0.053, 0.1 ]  TimeConstants6=[]  TimeConstants7=[]  TimeConstants8=[]  StatorResistance=2.8544e-3  Mechanical="[ 3.2  0  32]"  PolePairs=32  InitialConditions=[0 -67.6291 0.902477 0.902477 0.902477 -4.2812 -124.281 115.719 1.45511]  SetSaturation=off  Saturation=[0.6404,0.7127,0.8441,0.9214,0.9956,1.082,1.19,1.316,1.457;0.7,0.7698,0.8872,0.9466,0.9969,1.046,1.1,1.151,1.201]  LoadFlowParameters=[1 180000000 0 0 0]  TsPowergui=0  TsBlock=-1  IterativeModel=Trapezoidal non iterative  IterativeDiscreteModel=Trapezoidal non iterative  BusType=PV  Pref=180000000  Qref=0  Qmin=-Inf  Qmax=Inf  PLF=0  QLF=0
  LG3_2200 MVA : spsSynchronousMachinepuStandardLib/Synchronous Machine pu Standard  PresetModel=No  MechanicalLoad=Mechanical power Pm  ShowDetailedParameters=on  RotorType=Salient-pole  Units=per unit standard parameters  MeasurementBus=off  NominalParameters="[2200E6  13800   60 ]"  Reactances1=[ 31 32 33 34 35 36 37 ]  Reactances2=[ 1.305, 0.296, 0.252, 0.474, 0.243, 0.18 ]  dAxisTimeConstants=Short-circuit  qAxisTimeConstants=Open-circuit  TimeConstants1=[]  TimeConstants2=[]  TimeConstants3=[]  TimeConstants4=[]  TimeConstants5=[ 1.01, 0.053, 0.1 ]  TimeConstants6=[]  TimeConstants7=[]  TimeConstants8=[]  StatorResistance=2.8544e-3  Mechanical="[ 3.2  0  32]"  PolePairs=32  InitialConditions=[0 -70.0065 0.820496 0.820496 0.820496 -4.90643 -124.906 115.094 1.38903]  SetSaturation=off  Saturation=[0.6404,0.7127,0.8441,0.9214,0.9956,1.082,1.19,1.316,1.457;0.7,0.7698,0.8872,0.9466,0.9969,1.046,1.1,1.151,1.201]  LoadFlowParameters=[1 1800000000 0 0 0]  TsPowergui=0  TsBlock=-1  IterativeModel=Trapezoidal non iterative  IterativeDiscreteModel=Trapezoidal non iterative  BusType=PV  Pref=1800000000  Qref=0  Qmin=-Inf  Qmax=Inf  PLF=0  QLF=0
  LG4 660 Mvar : spsThreePhaseSeriesRLCLoadLib/Three-Phase Series RLC Load  LConnTagsString=A|B|C  Configuration=Y (grounded)  NominalVoltage=735e3  Vabc=[1e3 1e3 1e3]  Vabcp=[1e3 1e3 1e3]  NominalFrequency=60  UnbalancedPower=off  ActivePower=2200000  InductivePower=660e6  CapacitivePower=0  Pabc=[10e3 9e3 11e3]  QLabc=[100 90 110]  QCabc=[100 90 110]  Pabcp=[10e3 9e3 11e3]  QLabcp=[100 90 110]  QCabcp=[100 90 110]  Measurements=None  LoadType=constant Z
  LG4-2700 MVA : spsSynchronousMachinepuStandardLib/Synchronous Machine pu Standard  PresetModel=No  MechanicalLoad=Mechanical power Pm  ShowDetailedParameters=on  RotorType=Salient-pole  Units=per unit standard parameters  MeasurementBus=off  NominalParameters="[2700E6  13800   60 ]"  Reactances1=[ 31 32 33 34 35 36 37 ]  Reactances2=[ 1.305, 0.296, 0.252, 0.474, 0.243, 0.18 ]  dAxisTimeConstants=Short-circuit  qAxisTimeConstants=Open-circuit  TimeConstants1=[]  TimeConstants2=[]  TimeConstants3=[]  TimeConstants4=[]  TimeConstants5=[ 1.01, 0.053, 0.1 ]  TimeConstants6=[]  TimeConstants7=[]  TimeConstants8=[]  StatorResistance=2.8544e-3  Mechanical="[ 3.7  0  32]"  PolePairs=32  InitialConditions=[0 -69.506 0.926038 0.926038 0.926038 -2.40174 -122.402 117.598 1.38766]  SetSaturation=off  Saturation=[0.6404,0.7127,0.8441,0.9214,0.9956,1.082,1.19,1.316,1.457;0.7,0.7698,0.8872,0.9466,0.9969,1.046,1.1,1.151,1.201]  LoadFlowParameters=[1 2500000000 0 0 0]  TsPowergui=0  TsBlock=-1  IterativeModel=Trapezoidal non iterative  IterativeDiscreteModel=Trapezoidal non iterative  BusType=PV  Pref=2500000000  Qref=0  Qmin=-Inf  Qmax=Inf  PLF=0  QLF=0
  LG4-LMO 3*118km : spsDistributedParametersLineLib/Distributed Parameters Line  Phases=3  Length=118  Frequency=60  Resistance="[0.01273  0.3864]/3"  Inductance="[0.9337e-3  4.1264e-3]/3"  Capacitance=[12.74e-9 7.751e-9]*3  x1=[-0.000675 -9.12415791991974e-10 446066.324942421 -570785.422694355;-0.0006 -9.69770022108942e-10 462024.453036346 -557946.70660757;-0.000525 -1.02634903290822e-09 477613.245851725 -544661.976460394;-0.00045 -1.08210759599425e-09 492820.241946097 -530941.851862843;-0.000375 -1.13700113882485e-09 507633.285079461 -516797.300472596;-0.0003 -1.19098578034177e-09 522040.533931782 -502239.629227615;-0.000225 -1.24401836604858e-09 536030.471568765 -487280.475307553;-0.00015 -1.29605650250769e-09 549591.914648318 -471931.796831172;-7.5e-05 -1.34705859122902e-09 562714.022360339 -456205.863297203]  x2=[-0.000675 4.38355081359327e-09 414813.875448564 -602860.773674946;-0.0006 4.34006885285521e-09 431691.280998691 -590892.755025049;-0.000525 4.29311750748146e-09 448223.599143885 -578452.385747747;-0.00045 4.24273430965912e-09 464397.614201975 -565549.610483897;-0.000375 4.18895953494566e-09 480200.396912793 -552194.743514625;-0.0003 4.13183617007319e-09 495619.314773631 -538398.460516251;-0.000225 4.07140987858558e-09 510642.04213747 -524171.790026312;-0.00015 4.00772896433569e-09 525256.570065909 -509526.104627524;-7.5e-05 3.94084433287201e-09 539451.215928932 -494473.111856707]  x3=[-0.000675 9.50081627505204e-12 2040.14143601564 -4504.23210447455;-0.0006 1.16075811175619e-11 2166.66257243603 -4444.75566914955;-0.000525 1.37050670373283e-11 2291.45171194706 -4381.72616414968;-0.00045 1.57915973361997e-11 2414.40910001996 -4315.19397429684;-0.000375 1.786550407378e-11 2535.43644639999 -4245.21228440563;-0.0003 1.99251294007551e-11 2654.43700367825 -4171.8370367682;-0.000225 2.1968826884152e-11 2771.31564463002 -4095.12688643482;-0.00015 2.3994962823472e-11 2885.97893825802 -4015.14315432596;-7.5e-05 2.60019175566461e-11 2998.33522447974 -3931.94977821329]  x4=[-0.000675 6.64680002136731e-12 6463.18076750012 -9178.7845674661;-0.0006 4.04075494158341e-12 6720.08725258081 -8992.39755657614;-0.000525 1.43147974412483e-12 6971.62180273258 -8798.82216066774;-0.00045 -1.17893975633882e-12 7217.58334508463 -8598.2131209506;-0.000375 -3.78841683039965e-12 7457.77526174335 -8390.73080122165;-0.0003 -6.39486550201097e-12 7692.00554696562 -8176.54105967268;-0.000225 -8.99620221598471e-12 7920.08696064528 -7955.81511630589;-0.00015 -1.15903475035535e-11 8141.83717798999 -7728.72941606317;-7.5e-05 -1.41752276446662e-11 8357.0789352689 -7495.46548777878]  x5=0.000667339049054976  V1=ones(3,3)  V2=ones(3,3)  I1=ones(3,3)  I2=ones(3,3)  nHarmo=1  Measurements=None  Decoupling=on  VsMag0=[591479.207020584 591478.775968394 591479.558478697]  VrMag0=[597501.49549937 597500.918482429 597501.873521745]  VsAngle0=[22.5874691411725 -97.41246743921 142.587537012216]  VrAngle0=[19.1109154470794 -100.889010750024 139.111000266937]  IsMag0=[4048.55267184926 4048.55521766134 4048.56794769796]  IrMag0=[9191.46117506309 9191.44543051311 9191.45421674771]  IsAngle0=[8.94759792225275 -111.052173248457 128.947681135238]  IrAngle0=[19.7310305258253 -100.268962895628 139.731118811253]
      settings: AttributesFormatString=\n  LibrarySourceBlock=sps_lib/Power Grid Elements/Distributed Parameters Line
  LMO 330 Mvar : spsThreePhaseSeriesRLCLoadLib/Three-Phase Series RLC Load  LConnTagsString=A|B|C  Configuration=Y (grounded)  NominalVoltage=735e3  Vabc=[1e3 1e3 1e3]  Vabcp=[1e3 1e3 1e3]  NominalFrequency=60  UnbalancedPower=off  ActivePower=1100000  InductivePower=330e6  CapacitivePower=0  Pabc=[10e3 9e3 11e3]  QLabc=[100 90 110]  QCabc=[100 90 110]  Pabcp=[10e3 9e3 11e3]  QLabcp=[100 90 110]  QCabcp=[100 90 110]  Measurements=None  LoadType=constant Z
  LMO-ALB 3*218km : spsDistributedParametersLineLib/Distributed Parameters Line  Phases=3  Length=218  Frequency=60  Resistance="[0.01273  0.3864]/3"  Inductance="[0.9337e-3  4.1264e-3]/3"  Capacitance=[12.74e-9 7.751e-9]*3  x1=[-0.001275 4.6029317992722e-09 0 0;-0.0012 4.58821800295725e-09 0 0;-0.001125 4.56983645537282e-09 0 0;-0.00105 4.54780185044681e-09 0 0;-0.000975 4.52213180230526e-09 0 0;-0.0009 4.49284683119188e-09 0 0;-0.000825 4.45997034706451e-09 380078.033365231 -625341.876126177;-0.00075 4.42352863088152e-09 397604.874033269 -614346.874646447;-0.000675 4.38355081359327e-09 414813.875448564 -602860.773674946;-0.0006 4.34006885285521e-09 431691.280998691 -590892.755025049;-0.000525 4.29311750748146e-09 448223.599143885 -578452.385747747;-0.00045 4.24273430965912e-09 464397.614201975 -565549.610483897;-0.000375 4.18895953494566e-09 480200.396912793 -552194.743514625;-0.0003 4.13183617007319e-09 495619.314773631 -538398.460516251;-0.000225 4.07140987858558e-09 510642.04213747 -524171.790026312;-0.00015 4.00772896433569e-09 525256.570065909 -509526.104627524;-7.5e-05 3.94084433287201e-09 539451.215928932 -494473.111856707]  x2=[-0.001275 1.65591356558967e-08 0 0;-0.0012 1.65943408488805e-08 0 0;-0.001125 1.66162807796916e-08 0 0;-0.00105 1.6624937909885e-08 0 0;-0.000975 1.66203053190834e-08 0 0;-0.0009 1.66023867105088e-08 0 0;-0.000825 1.6571196408023e-08 256317.712946208 -689303.96475024;-0.00075 1.65267593446763e-08 275702.267037867 -681782.177055613;-0.000675 1.64691110427775e-08 294866.428955643 -673715.383120265;-0.0006 1.63982975854968e-08 313794.879161719 -665110.031415841;-0.000525 1.63143755800288e-08 332472.486542616 -655973.000928828;-0.00045 1.62174121123403e-08 350884.32050477 -646311.595661597;-0.000375 1.6107484693544e-08 369015.662909823 -636133.538793692;-0.0003 1.59846811979364e-08 386852.019840075 -625446.966508046;-0.000225 1.5849099792753e-08 404379.133184701 -614260.421487032;-0.00015 1.57008488596947e-08 421582.992037467 -602582.846083581;-7.5e-05 1.55400469082889e-08 438449.843896835 -590423.575172798]  x3=[-0.001275 2.78863735028711e-11 0 0;-0.0012 3.08249653493774e-11 0 0;-0.001125 3.37389161902213e-11 0 0;-0.00105 3.66258966576854e-11 0 0;-0.000975 3.94835989437564e-11 0 0;-0.0009 4.23097386449511e-11 0 0;-0.000825 4.51020565884337e-11 504.220647789621 -2691.25110183665;-0.00075 4.78583206379641e-11 580.102277876931 -2675.9203491071;-0.000675 5.05763274782334e-11 655.520183079169 -2658.45050659342;-0.0006 5.32539043761603e-11 730.414075476848 -2638.85553942043;-0.000525 5.5888910917741e-11 804.724086038301 -2617.15111150508;-0.00045 5.84792407190631e-11 878.390812478067 -2593.35457303494;-0.000375 6.10228231101167e-11 951.355366742167 -2567.48494659877;-0.0003 6.35176247900567e-11 1023.55942208232 -2539.56291198013;-0.000225 6.59616514525917e-11 1094.94525968144 -2509.61078962626;-0.00015 6.83529493802025e-11 1165.4558147932 -2477.65252280551;-7.5e-05 7.06896070059141e-11 1235.03472235869 -2443.71365846737]  x4=[-0.001275 5.54768834450226e-11 0 0;-0.0012 5.32343808997036e-11 0 0;-0.001125 5.09493236048066e-11 0 0;-0.00105 4.86235382001708e-11 0 0;-0.000975 4.62588838830628e-11 0 0;-0.0009 4.38572509219634e-11 0 0;-0.000825 4.14205591455154e-11 4425.69676226945 -12765.9262438942;-0.00075 3.89507564078422e-11 4784.82745779799 -12635.7066271848;-0.000675 3.64498170314632e-11 5140.13323546709 -12495.3862199304;-0.0006 3.39197402290502e-11 5491.33006927442 -12345.0771921176;-0.000525 3.13625485052875e-11 5838.13721784455 -12184.8996984834;-0.00045 2.87802860401127e-11 6180.27744884923 -12014.9817824655;-0.000375 2.61750170546306e-11 6517.47726062271 -11835.4592738461;-0.0003 2.35488241610063e-11 6849.46710079479 -11646.4756801717;-0.000225 2.09038066976567e-11 7175.98158176687 -11448.1820720357;-0.00015 1.8242079051072e-11 7496.75969285867 -11240.7369623143;-7.5e-05 1.5565768965607e-11 7811.54500895628 -11024.3061794544]  x5=0.00123288061605072  V1=ones(3,3)  V2=ones(3,3)  I1=ones(3,3)  I2=ones(3,3)  nHarmo=1  Measurements=None  Decoupling=on  VsMag0=[597501.49549937 597500.918482429 597501.873521745]  VrMag0=[600465.939453852 600465.308790857 600466.091594043]  VsAngle0=[19.1109154470794 -100.889010750024 139.111000266937]  VrAngle0=[8.21765611494233 -111.782292378922 128.217733982922]  IsMag0=[2247.12525868881 2247.11361990981 2247.1220088738]  IrMag0=[11088.6272022732 11088.6249727979 11088.6349972326]  IsAngle0=[-1.56829194732943 -121.568216294825 118.432002879358]  IrAngle0=[6.94042447158262 -113.059522369363 126.940461027599]
      settings: AttributesFormatString=\n  LibrarySourceBlock=sps_lib/Power Grid Elements/Distributed Parameters Line
  LMO7 : spsThreePhaseVIMeasurementLib/Three-Phase V-I Measurement  VoltageMeasurement=no  SetLabelV=on  LabelV=Vabc_LMO7  Vpu=on  VpuLL=off  CurrentMeasurement=no  SetLabelI=off  LabelI=A1  Ipu=off  Pbase=100e6  Vbase=735e3  OutputType=Magnitude  PhasorSimulation=off  PSBequivalent=0
  LVD 990 Mvar : spsThreePhaseSeriesRLCLoadLib/Three-Phase Series RLC Load  LConnTagsString=A|B|C  Configuration=Y (grounded)  NominalVoltage=735e3  Vabc=[1e3 1e3 1e3]  Vabcp=[1e3 1e3 1e3]  NominalFrequency=60  UnbalancedPower=off  ActivePower=3300000  InductivePower=990e6  CapacitivePower=0  Pabc=[10e3 9e3 11e3]  QLabc=[100 90 110]  QCabc=[100 90 110]  Pabcp=[10e3 9e3 11e3]  QLabcp=[100 90 110]  QCabcp=[100 90 110]  Measurements=None  LoadType=constant Z
  LVD-MTL 3*260km : spsDistributedParametersLineLib/Distributed Parameters Line  Phases=3  Length=260  Frequency=60  Resistance="[0.01273  0.3864]/3"  Inductance="[0.9337e-3  4.1264e-3]/3"  Capacitance=[12.74e-9 7.751e-9]*3  x1=[-0.0015 5.6474908312105e-08 -89258.2599346528 -744297.731345168;-0.001425 5.66820717477919e-08 -68180.8722481852 -746523.607859629;-0.00135 5.68439244025883e-08 -47048.9818156449 -748152.724824162;-0.001275 5.69603368939585e-08 -25879.4811469147 -749183.77994759;-0.0012 5.70312161635381e-08 -4689.29281692486 -749615.949020224;-0.001125 5.70565055515234e-08 16504.6440619942 -749448.886572721;-0.00105 5.70361848419646e-08 37685.3873809795 -748682.726152243;-0.000975 5.69702702789261e-08 58836.0055778984 -747318.08021571;-0.0009 5.68588145535009e-08 79939.5911721792 -745356.039640201;-0.000825 5.67019067616908e-08 100979.274280394 -742798.172850935;-0.00075 5.64996723331835e-08 121938.236101783 -739646.524567484;-0.000675 5.62522729310872e-08 142799.722362951 -735903.614169266;-0.0006 5.59599063226983e-08 163547.05671097 -731572.433681583;-0.000525 5.56228062214104e-08 184163.654044209 -726656.44538385;-0.00045 5.52412420998865e-08 204633.033770203 -721159.579041892;-0.000375 5.48155189746473e-08 224938.832979991 -715086.22876656;-0.0003 5.43459771622454e-08 245064.819528375 -708441.249501139;-0.000225 5.38329920072213e-08 264994.905009646 -701229.953140381;-0.00015 5.3276973582059e-08 284713.157618409 -693458.10428426;-7.5e-05 5.26783663593803e-08 304203.81488523 -685131.915629839]  x2=[-0.0015 8.73198516027194e-08 -318141.458272012 -654659.491566303;-0.001425 8.75226112219733e-08 -299506.6986917 -663391.865920958;-0.00135 8.76554066049572e-08 -280632.518039061 -671593.934968232;-0.001275 8.77181315970738e-08 -261534.004045322 -679259.142099624;-0.0012 8.77107360569241e-08 -242226.423770354 -686381.359865835;-0.001125 8.76332258963897e-08 -222725.211398413 -692954.894874956;-0.00105 8.74856630759072e-08 -203045.955900289 -698974.492343679;-0.000975 8.72681655549372e-08 -183204.388571726 -704435.340297891;-0.0009 8.69809071976704e-08 -163216.370458061 -709333.073419292;-0.000825 8.66241176340422e-08 -143097.879675145 -713663.77653496;-0.00075 8.61980820761709e-08 -122864.998636688 -717423.987747089;-0.000675 8.57031410903627e-08 -102533.901198218 -720610.701200368;-0.0006 8.51396903248689e-08 -82120.8397279515 -723221.369484821;-0.000525 8.45081801936104e-08 -61642.1321148977 -725253.905672165;-0.00045 8.38091155161236e-08 -41114.1487245874 -726706.684984072;-0.000375 8.30430551140157e-08 -20553.2993128542 -727578.546090988;-0.0003 8.2210611364251e-08 23.9800918736146 -727868.792040484;-0.000225 8.13124497096263e-08 20601.2403272829 -727577.190814389;-0.00015 8.03492881268259e-08 41162.0322463841 -726703.975514261;-7.5e-05 7.93218965524822e-08 61689.9198667078 -725249.844175051]  x3=[-0.0015 2.45706558582318e-10 326.034617914444 -307.945403567002;-0.001425 2.54185405084449e-10 334.610417599536 -298.604572740696;-0.00135 2.62461059662923e-10 342.91873483651 -289.025041987744;-0.001275 2.70526906886092e-10 350.952928083688 -279.214469038459;-0.0012 2.78376499039096e-10 358.706574929916 -269.180696314749;-0.001125 2.86003561278072e-10 366.17347722854 -258.931744661008;-0.00105 2.93401996646163e-10 373.347666052109 -248.475806932373;-0.000975 3.00565890947336e-10 380.223406463847 -237.821241445484;-0.0009 3.07489517474098e-10 386.795202102071 -226.97656529697;-0.000825 3.14167341585339e-10 393.0577995739 -215.950447555016;-0.00075 3.20594025130638e-10 399.006192654736 -204.751702329439;-0.000675 3.26764430717501e-10 404.635626290162 -193.389281725826;-0.0006 3.32673625818112e-10 409.941600397065 -181.872268689357;-0.000525 3.38316886712321e-10 414.919873460928 -170.209869744036;-0.00045 3.43689702263714e-10 419.566465926432 -158.41140763314;-0.000375 3.48787777525746e-10 423.877663378658 -146.486313866758;-0.0003 3.53607037175056e-10 427.850019512324 -134.444121182387;-0.000225 3.58143628769217e-10 431.480358886716 -122.294455924607;-0.00015 3.62393925826321e-10 434.765779464086 -110.047030349928;-7.5e-05 3.66354530723933e-10 437.703654929492 -97.7116348629642]  x4=[-0.0015 2.65776478171551e-10 -7428.61939570882 -14286.1681180435;-0.001425 2.63147341161606e-10 -7021.77252832359 -14490.4696992907;-0.00135 2.60307848193426e-10 -6609.31256341595 -14683.1878207719;-0.001275 2.57260269114245e-10 -6191.56921517098 -14864.1684265695;-0.0012 2.54007040112147e-10 -5768.87642122959 -15033.2668435563;-0.001125 2.50550761768621e-10 -5341.57207574384 -15190.3478970451;-0.00105 2.46894196979693e-10 -4909.99775926953 -15335.2860188451;-0.000975 2.43040268747308e-10 -4474.49846571195 -15467.9653476393;-0.0009 2.38992057842726e-10 -4035.422326543 -15588.2798216025;-0.000825 2.34752800343807e-10 -3593.12033251024 -15696.133263185;-0.00075 2.3032588504813e-10 -3147.94605306026 -15791.4394559957;-0.000675 2.25714850764051e-10 -2700.25535370065 -15874.1222137225;-0.0006 2.20923383481823e-10 -2250.40611152659 -15944.1154410338;-0.000525 2.15955313427082e-10 -1798.75792913934 -16001.3631864147;-0.00045 2.10814611999013e-10 -1345.67184718545 -16045.8196868935;-0.000375 2.05505388595685e-10 -891.5100557464 -16077.4494046238;-0.0003 2.00031887329051e-10 -436.635604809343 -16096.2270552933;-0.000225 1.94398483632277e-10 18.5878859494503 -16102.1376283353;-0.00015 1.88609680762083e-10 473.79651783662 -16095.1763989282;-7.5e-05 1.82670106198914e-10 928.62640403676 -16075.3489317723]  x5=0.00147040807418893  V1=ones(3,3)  V2=ones(3,3)  I1=ones(3,3)  I2=ones(3,3)  nHarmo=1  Measurements=None  Decoupling=on  VsMag0=[612070.919184233 612070.526870855 612070.832121117]  VrMag0=[594302.51828106 594302.52559147 594302.380387351]  VsAngle0=[-4.43840982431121 -124.438398032275 115.561627875921]  VrAngle0=[-23.5181046799956 -143.518120437643 96.4818868308235]  IsMag0=[368.438417399341 368.422778584527 368.434712931915]  IrMag0=[13227.9520808222 13227.9561692155 13227.9649229573]  IsAngle0=[49.0336389584917 -70.9656221607441 169.036114576136]  IrAngle0=[-25.0738913250262 -145.073837319252 94.9261203418385]
      settings: AttributesFormatString=\n  LibrarySourceBlock=sps_lib/Power Grid Elements/Distributed Parameters Line
  LVD7 : spsThreePhaseVIMeasurementLib/Three-Phase V-I Measurement  VoltageMeasurement=no  SetLabelV=on  LabelV=Vabc_LVD7  Vpu=on  VpuLL=off  CurrentMeasurement=no  SetLabelI=off  LabelI=A1  Ipu=off  Pbase=100e6  Vbase=735e3  OutputType=Magnitude  PhasorSimulation=off  PSBequivalent=0
  Load Flow Bus1 : spsLoadFlowBusLib/Load Flow Bus  LConnTagsString=a  Phases=single  Connectors=on one side  ID=LG31_13.8  Vbase=13.8e3  Vref=1  Vangle=0  VLF=1  VLFb=1  VLFc=1  angleLF=-0.0351  angleLFb=0  angleLFc=0
      settings: AttributesFormatString=%<ID>\n%<Vbase>V\n%<VLF>pu\n%<angleLF>deg.
  Load Flow Bus10 : spsLoadFlowBusLib/Load Flow Bus  LConnTagsString=a  Phases=single  Connectors=on one side  ID=LVD7  Vbase=735e3  Vref=1  Vangle=0  VLF=1.05  VLFb=1  VLFc=1  angleLF=-12.02  angleLFb=0  angleLFc=0
      settings: AttributesFormatString=%<ID>\n%<Vbase>V\n%<VLF>pu\n%<angleLF>deg.
  Load Flow Bus11 : spsLoadFlowBusLib/Load Flow Bus  LConnTagsString=a  Phases=single  Connectors=on one side  ID=CHM7  Vbase=735e3  Vref=1  Vangle=0  VLF=1.047  VLFb=1  VLFc=1  angleLF=-4.064  angleLFb=0  angleLFc=0
      settings: AttributesFormatString=%<ID>\n%<Vbase>V\n%<VLF>pu\n%<angleLF>deg.
  Load Flow Bus12 : spsLoadFlowBusLib/Load Flow Bus  LConnTagsString=a  Phases=single  Connectors=on one side  ID=LG47  Vbase=735e3  Vref=1  Vangle=0  VLF=1.004  VLFb=1  VLFc=1  angleLF=20.71  angleLFb=0  angleLFc=0
      settings: AttributesFormatString=%<ID>\n%<Vbase>V\n%<VLF>pu\n%<angleLF>deg.
  Load Flow Bus2 : spsLoadFlowBusLib/Load Flow Bus  LConnTagsString=a  Phases=single  Connectors=on one side  ID=LG3_13.8  Vbase=13.8e3  Vref=1  Vangle=0  VLF=1  VLFb=1  VLFc=1  angleLF=-0.6025  angleLFb=0  angleLFc=0
      settings: AttributesFormatString=%<ID>\n%<Vbase>V\n%<VLF>pu\n%<angleLF>deg.
  Load Flow Bus3 : spsLoadFlowBusLib/Load Flow Bus  LConnTagsString=a  Phases=single  Connectors=on one side  ID=LG4_13.8  Vbase=13.8e3  Vref=1  Vangle=0  VLF=1  VLFb=1  VLFc=1  angleLF=-3.293  angleLFb=0  angleLFc=0
      settings: AttributesFormatString=%<ID>\n%<Vbase>V\n%<VLF>pu\n%<angleLF>deg.
  Load Flow Bus4 : spsLoadFlowBusLib/Load Flow Bus  LConnTagsString=a  Phases=single  Connectors=on one side  ID=LG2_13.8  Vbase=13.8e3  Vref=1  Vangle=0  VLF=1  VLFb=1  VLFc=1  angleLF=0  angleLFb=0  angleLFc=0
      settings: AttributesFormatString=%<ID>\n%<Vbase>V\n%<VLF>pu\n%<angleLF>deg.
  Load Flow Bus5 : spsLoadFlowBusLib/Load Flow Bus  LConnTagsString=a  Phases=single  Connectors=on one side  ID=LG27  Vbase=735e3  Vref=1  Vangle=0  VLF=1  VLFb=1  VLFc=1  angleLF=23.57  angleLFb=0  angleLFc=0
      settings: AttributesFormatString=%<ID>\n%<Vbase>V\n%<VLF>pu\n%<angleLF>deg.
  Load Flow Bus6 : spsLoadFlowBusLib/Load Flow Bus  LConnTagsString=a  Phases=single  Connectors=on one side  ID=LG37  Vbase=735e3  Vref=1  Vangle=0  VLF=0.994  VLFb=1  VLFc=1  angleLF=24.1  angleLFb=0  angleLFc=0
      settings: AttributesFormatString=%<ID>\n%<Vbase>V\n%<VLF>pu\n%<angleLF>deg.
  Load Flow Bus7 : spsLoadFlowBusLib/Load Flow Bus  LConnTagsString=a  Phases=single  Connectors=on one side  ID=LMO7  Vbase=735e3  Vref=1  Vangle=0  VLF=1.016  VLFb=1  VLFc=1  angleLF=17.31  angleLFb=0  angleLFc=0
      settings: AttributesFormatString=%<ID>\n%<Vbase>V\n%<VLF>pu\n%<angleLF>deg.
  Load Flow Bus8 : spsLoadFlowBusLib/Load Flow Bus  LConnTagsString=a  Phases=single  Connectors=on one side  ID=NEM_ALB7  Vbase=735e3  Vref=1  Vangle=0  VLF=1.028  VLFb=1  VLFc=1  angleLF=8.928  angleLFb=0  angleLFc=0
      settings: AttributesFormatString=%<ID>\n%<Vbase>V\n%<VLF>pu\n%<angleLF>deg.
  Load Flow Bus9 : spsLoadFlowBusLib/Load Flow Bus  LConnTagsString=a  Phases=single  Connectors=on one side  ID=ABI_CHB7  Vbase=735e3  Vref=1  Vangle=0  VLF=1.046  VLFb=1  VLFc=1  angleLF=0.1334  angleLFb=0  angleLFc=0
      settings: AttributesFormatString=%<ID>\n%<Vbase>V\n%<VLF>pu\n%<angleLF>deg.
  NEM-ABI 6*236 : spsDistributedParametersLineLib/Distributed Parameters Line  Phases=3  Length=236  Frequency=60  Resistance="[0.01273  0.3864]/6"  Inductance="[0.9337e-3  4.1264e-3]/6"  Capacitance=[12.74e-9 7.751e-9]*6  x1=[-0.00135 1.58511888278563e-08 0 0;-0.001275 1.59130465440801e-08 0 0;-0.0012 1.59621836143743e-08 0 0;-0.001125 1.59985607593168e-08 0 0;-0.00105 1.60221488995744e-08 0 0;-0.000975 1.60329291791489e-08 0 0;-0.0009 1.60308929804496e-08 0 0;-0.000825 1.60160419311825e-08 284117.477880549 -680689.106291918;-0.00075 1.59883879030494e-08 303247.373018692 -672384.845536947;-0.000675 1.59479530022571e-08 322134.856846686 -663543.090624288;-0.0006 1.58947695518467e-08 340764.830998944 -654170.909517533;-0.000525 1.58288800658546e-08 359122.402959179 -644275.794194861;-0.00045 1.57503372153279e-08 377192.897965245 -633865.654660059;-0.000375 1.56592037862195e-08 394961.870739922 -622948.812619392;-0.0003 1.55555526291982e-08 412415.11703825 -611533.994829353;-0.000225 1.54394666014131e-08 429538.685002179 -599630.326120632;-0.00015 1.53110385002586e-08 446318.886313481 -587247.322103861;-7.5e-05 1.51703709891938e-08 462742.307135971 -574394.881562986]  x2=[-0.00135 2.8534306575093e-08 0 0;-0.001275 2.86036619672485e-08 0 0;-0.0012 2.86501520296781e-08 0 0;-0.001125 2.86737395989373e-08 0 0;-0.00105 2.86744058194839e-08 0 0;-0.000975 2.86521501587516e-08 0 0;-0.0009 2.86069904075749e-08 0 0;-0.000825 2.85389626659681e-08 125357.104453978 -735061.346284793;-0.00075 2.84481213142669e-08 146087.597415325 -731223.617196845;-0.000675 2.83345389696579e-08 166701.310186514 -726801.359137407;-0.0006 2.81983064281295e-08 187181.764480956 -721798.107191908;-0.000525 2.80395325918911e-08 207512.588536848 -716217.860883402;-0.00045 2.78583443823179e-08 227677.530204513 -710065.080975406;-0.000375 2.76548866384925e-08 247660.469938116 -703344.685906038;-0.0003 2.74293220014222e-08 267445.433681382 -696062.047856291;-0.000225 2.71818307840267e-08 287016.605637016 -688222.988455595;-0.00015 2.69126108269983e-08 306358.340909605 -679833.774128092;-7.5e-05 2.66218773406517e-08 325455.17801191 -670901.111083357]  x3=[-0.00135 1.51740118550679e-10 0 0;-0.001275 1.58664468230525e-10 0 0;-0.0012 1.65461983962117e-10 0 0;-0.001125 1.72127231915382e-10 0 0;-0.00105 1.78654883993088e-10 0 0;-0.000975 1.85039722090043e-10 0 0;-0.0009 1.91276642264361e-10 0 0;-0.000825 1.97360658817483e-10 -448.187482110444 -4499.57322109266;-0.00075 2.03286908279667e-10 -320.801895603415 -4510.44404859478;-0.000675 2.09050653297765e-10 -193.159864969475 -4517.70929613657;-0.0006 2.146472864222e-10 -65.363425294923 -4521.36315599029;-0.000525 2.20072333790082e-10 62.4852649017157 -4521.40270731629;-0.00045 2.25321458701552e-10 190.284005333649 -4517.82791849785;-0.000375 2.3039046508647e-10 317.930635643161 -4510.64164716644;-0.0003 2.35275300858691e-10 445.323117067042 -4499.84963791742;-0.000225 2.39972061155237e-10 572.359614004811 -4485.46051771785;-0.00015 2.44476991457792e-10 698.938575424541 -4467.48578901027;-7.5e-05 2.48786490593999e-10 824.958816041196 -4445.93982051778]  x4=[-0.00135 1.68347305508067e-10 0 0;-0.001275 1.64905790689492e-10 0 0;-0.0012 1.61332452704983e-10 0 0;-0.001125 1.57630148026251e-10 0 0;-0.00105 1.5380183621901e-10 0 0;-0.000975 1.49850577577141e-10 0 0;-0.0009 1.45779530676349e-10 0 0;-0.000825 1.41591949849235e-10 4622.22438525001 -28011.6084746931;-0.00075 1.37291182583841e-10 5412.27949589078 -27869.7398149522;-0.000675 1.32880666847715e-10 6198.00811311319 -27705.5925116245;-0.0006 1.28363928339654e-10 6978.78213748269 -27519.2977815528;-0.000525 1.23744577671312e-10 7753.97743019042 -27311.0045458939;-0.00045 1.19026307480935e-10 8522.9743119803 -27080.8793110734;-0.000375 1.14212889481521e-10 9285.15805851105 -26829.106035683;-0.0003 1.09308171445771e-10 10039.9193917575 -26555.8859834267;-0.000225 1.04316074130239e-10 10786.6549670581 -26261.437562234;-0.00015 9.92405881411366e-11 11524.7678554194 -25945.9961496675;-7.5e-05 9.40857707443061e-11 12253.668020692 -25609.813904766]  x5=0.00133467809810995  V1=ones(3,3)  V2=ones(3,3)  I1=ones(3,3)  I2=ones(3,3)  nHarmo=1  Measurements=None  Decoupling=on  VsMag0=[602251.717194481 602251.086049773 602251.913986722]  VrMag0=[608840.309919382 608839.972623117 608840.270927256]  VsAngle0=[10.4755045319416 -109.524439183 130.475584674536]  VrAngle0=[-2.5019024195443 -122.501888330518 117.498132114124]  IsMag0=[3712.64388955984 3712.61521802381 3712.6059745509]  IrMag0=[23309.6118788358 23309.6245706238 23309.648848921]  IsAngle0=[-17.8678983044052 -137.868318490117 102.132274803425]  IrAngle0=[-2.81003503241263 -122.809948112052 117.18998141058]
      settings: AttributesFormatString=\n  LibrarySourceBlock=sps_lib/Power Grid Elements/Distributed Parameters Line
  NEM-ALB 1980 Mvar : spsThreePhaseSeriesRLCLoadLib/Three-Phase Series RLC Load  LConnTagsString=A|B|C  Configuration=Y (grounded)  NominalVoltage=735e3  Vabc=[1e3 1e3 1e3]  Vabcp=[1e3 1e3 1e3]  NominalFrequency=60  UnbalancedPower=off  ActivePower=6600000  InductivePower=1980e6  CapacitivePower=0  Pabc=[10e3 9e3 11e3]  QLabc=[100 90 110]  QCabc=[100 90 110]  Pabcp=[10e3 9e3 11e3]  QLabcp=[100 90 110]  QCabcp=[100 90 110]  Measurements=None  LoadType=constant Z
  NEM-ALB7 : spsThreePhaseVIMeasurementLib/Three-Phase V-I Measurement  VoltageMeasurement=no  SetLabelV=on  LabelV=Vabc_NEM7  Vpu=on  VpuLL=off  CurrentMeasurement=no  SetLabelI=off  LabelI=A1  Ipu=off  Pbase=100e6  Vbase=735e3  OutputType=Magnitude  PhasorSimulation=off  PSBequivalent=0
  Regulators1 : Subsystem
  Regulators2 : Subsystem
  Regulators3 : Subsystem
  Regulators4 : Subsystem
  MTLa : PMIOPort  Side=Right
  MTLb : PMIOPort  Port=2  Side=Right
  MTLc : PMIOPort  Port=3  Side=Right
  CHM7a : PMIOPort  Port=4  Side=Right
  CHM7b : PMIOPort  Port=5  Side=Right
  CHM7c : PMIOPort  Port=6  Side=Right
  wires:
  Regulators2/1(Pm) -> LG3_2200 MVA/1
  Regulators4/2(Vf) -> LG4-2700 MVA/2
  Regulators4/1(Pm) -> LG4-2700 MVA/1
  Regulators3/2(Vf) -> LG31-200 MVA/2
  Regulators3/1(Pm) -> LG31-200 MVA/1
  Regulators2/2(Vf) -> LG3_2200 MVA/2
  LG3_2200 MVA/1 -> Regulators2/1(m)
  Regulators1/1(Pm) -> LG2_5500 MVA/1
  Regulators1/2(Vf) -> LG2_5500 MVA/2
  LG2_5500 MVA/1 -> Regulators1/1(m)
  LG31-200 MVA/1 -> Regulators3/1(m)
  LG4-2700 MVA/1 -> Regulators4/1(m)
  connections:
  LG2-NENI 3*279km/RConn1 -- "Cs NEM "/LConn1
  LG2-NENI 3*279km/RConn2 -- "Cs NEM "/LConn2
  LG2-NENI 3*279km/RConn3 -- "Cs NEM "/LConn3
  CHB-CHM 3*195km/RConn1 -- "Cs  CHMN "/LConn1
  CHB-CHM 3*195km/RConn2 -- "Cs  CHMN "/LConn2
  CHB-CHM 3*195km/RConn3 -- "Cs  CHMN "/LConn3
  Load Flow Bus2/LConn1 -- 2200 MVA 13.8 kV/735 kV/LConn1 -- LG3_2200 MVA/RConn1 -- 110 MW/LConn1
  2200 MVA 13.8 kV/735 kV/LConn2 -- LG3_2200 MVA/RConn2 -- 110 MW/LConn2
  2200 MVA 13.8 kV/735 kV/LConn3 -- LG3_2200 MVA/RConn3 -- 110 MW/LConn3
  Load Flow Bus1/LConn1 -- 200 MVA 13.8 kV/735 kV/LConn1 -- LG31-200 MVA/RConn1 -- 10 MW/LConn1
  200 MVA 13.8 kV/735 kV/LConn2 -- LG31-200 MVA/RConn2 -- 10 MW/LConn2
  200 MVA 13.8 kV/735 kV/LConn3 -- LG31-200 MVA/RConn3 -- 10 MW/LConn3
  Load Flow Bus6/LConn1 -- 2200 MVA 13.8 kV/735 kV/RConn1 -- 200 MVA 13.8 kV/735 kV/RConn1 -- LG3-LMO 104km/LConn1 -- LG3 660 Mvar/LConn1 -- LG2-LG3 155km/RConn1
  2200 MVA 13.8 kV/735 kV/RConn2 -- LG3 660 Mvar/LConn2 -- LG2-LG3 155km/RConn2 -- 200 MVA 13.8 kV/735 kV/RConn2 -- LG3-LMO 104km/LConn2
  LG3-LMO 104km/RConn1 -- LMO7/RConn1 -- LG4-LMO 3*118km/RConn1 -- LMO 330 Mvar/LConn1
  LG3-LMO 104km/RConn2 -- LMO7/RConn2 -- LG4-LMO 3*118km/RConn2 -- LMO 330 Mvar/LConn2
  LG3-LMO 104km/RConn3 -- LMO7/RConn3 -- LG4-LMO 3*118km/RConn3 -- LMO 330 Mvar/LConn3
  LG4-LMO 3*118km/LConn1 -- LG4 660 Mvar/LConn1 -- 2700 MVA 13.8 kV/735 kV/RConn1 -- Load Flow Bus12/LConn1
  LG4-LMO 3*118km/LConn2 -- 2700 MVA 13.8 kV/735 kV/RConn2 -- LG4 660 Mvar/LConn2
  LG4 660 Mvar/LConn3 -- 2700 MVA 13.8 kV/735 kV/RConn3 -- LG4-LMO 3*118km/LConn3
  Load Flow Bus3/LConn1 -- LG4-2700 MVA/RConn1 -- 2700 MVA 13.8 kV/735 kV/LConn1 -- 135 MW/LConn1
  LG4-2700 MVA/RConn2 -- 2700 MVA 13.8 kV/735 kV/LConn2 -- 135 MW/LConn2
  LG4-2700 MVA/RConn3 -- 2700 MVA 13.8 kV/735 kV/LConn3 -- 135 MW/LConn3
  Load Flow Bus4/LConn1 -- 5500 MVA 13.8 kV/735 kV/LConn1 -- LG2_5500 MVA/RConn1 -- 275 MW/LConn1
  5500 MVA 13.8 kV/735 kV/LConn2 -- LG2_5500 MVA/RConn2 -- 275 MW/LConn2
  LG2_5500 MVA/RConn3 -- 5500 MVA 13.8 kV/735 kV/LConn3 -- 275 MW/LConn3
  5500 MVA 13.8 kV/735 kV/RConn1 -- LG2-NENI 3*279km/LConn1 -- LG2-LG3 155km/LConn1 -- LG2 660 Mvar/LConn1 -- Load Flow Bus5/LConn1
  LG2-LG3 155km/LConn2 -- 5500 MVA 13.8 kV/735 kV/RConn2 -- LG2-NENI 3*279km/LConn2 -- LG2 660 Mvar/LConn2
  LG2-LG3 155km/LConn3 -- 5500 MVA 13.8 kV/735 kV/RConn3 -- LG2-NENI 3*279km/LConn3 -- LG2 660 Mvar/LConn3
  "Cs NEM "/RConn1 -- NEM-ALB7/LConn1 -- Cs ALB/RConn1
  "Cs NEM "/RConn2 -- NEM-ALB7/LConn2 -- Cs ALB/RConn2
  "Cs NEM "/RConn3 -- NEM-ALB7/LConn3 -- Cs ALB/RConn3
  LMO7/LConn1 -- LMO-ALB 3*218km/LConn1
  LMO7/LConn2 -- LMO-ALB 3*218km/LConn2
  Load Flow Bus7/LConn1 -- LMO7/LConn3 -- LMO-ALB 3*218km/LConn3
  Cs ALB/LConn1 -- LMO-ALB 3*218km/RConn1
  Cs ALB/LConn2 -- LMO-ALB 3*218km/RConn2
  Cs ALB/LConn3 -- LMO-ALB 3*218km/RConn3
  200 MVA 13.8 kV/735 kV/RConn3 -- LG3-LMO 104km/LConn3 -- LG3 660 Mvar/LConn3 -- LG2-LG3 155km/RConn3 -- 2200 MVA 13.8 kV/735 kV/RConn3
  Load Flow Bus8/LConn1 -- NEM-ABI 6*236/LConn1 -- NEM-ALB7/RConn1 -- NEM-ALB 1980 Mvar/LConn1
  NEM-ALB 1980 Mvar/LConn2 -- NEM-ALB7/RConn2 -- NEM-ABI 6*236/LConn2
  NEM-ALB 1980 Mvar/LConn3 -- NEM-ALB7/RConn3 -- NEM-ABI 6*236/LConn3
  NEM-ABI 6*236/RConn1 -- "Cs ABI+CHB "/LConn1
  NEM-ABI 6*236/RConn2 -- "Cs ABI+CHB "/LConn2
  NEM-ABI 6*236/RConn3 -- "Cs ABI+CHB "/LConn3
  "Cs ABI+CHB "/RConn1 -- ABI-CHB7/LConn1
  "Cs ABI+CHB "/RConn2 -- ABI-CHB7/LConn2
  "Cs ABI+CHB "/RConn3 -- ABI-CHB7/LConn3
  Load Flow Bus9/LConn1 -- ABI+CHB 1320 Mvar/LConn1 -- CHB-CHM 3*195km/LConn1 -- ABI-CHB 3*271km/LConn1 -- ABI-CHB7/RConn1
  ABI-CHB 3*271km/LConn2 -- ABI-CHB7/RConn2 -- ABI+CHB 1320 Mvar/LConn2 -- CHB-CHM 3*195km/LConn2
  ABI-CHB 3*271km/LConn3 -- ABI-CHB7/RConn3 -- ABI+CHB 1320 Mvar/LConn3 -- CHB-CHM 3*195km/LConn3
  ABI-CHB 3*271km/RConn1 -- "Cs LVDN "/LConn1
  ABI-CHB 3*271km/RConn2 -- "Cs LVDN "/LConn2
  ABI-CHB 3*271km/RConn3 -- "Cs LVDN "/LConn3
  "Cs LVDN "/RConn1 -- LVD7/LConn1
  "Cs LVDN "/RConn2 -- LVD7/LConn2
  "Cs LVDN "/RConn3 -- LVD7/LConn3
  "Cs LVDS "/LConn1 -- LVD 990 Mvar/LConn1 -- Load Flow Bus10/LConn1 -- LVD7/RConn1
  "Cs LVDS "/LConn2 -- LVD7/RConn2 -- LVD 990 Mvar/LConn2
  "Cs LVDS "/LConn3 -- LVD7/RConn3 -- LVD 990 Mvar/LConn3
  "Cs LVDS "/RConn1 -- LVD-MTL 3*260km/LConn1
  "Cs LVDS "/RConn2 -- LVD-MTL 3*260km/LConn2
  "Cs LVDS "/RConn3 -- LVD-MTL 3*260km/LConn3
  MTLa/RConn1 -- LVD-MTL 3*260km/RConn1
  MTLb/RConn1 -- LVD-MTL 3*260km/RConn2
  MTLc/RConn1 -- LVD-MTL 3*260km/RConn3
  "Cs  CHMN "/RConn1 -- CHM7/LConn1
  "Cs  CHMN "/RConn2 -- CHM7/LConn2
  "Cs  CHMN "/RConn3 -- CHM7/LConn3
  CHM 1320Mvar/LConn2 -- CHM7/RConn2 -- CHM7b/RConn1
  Load Flow Bus11/LConn1 -- CHM 1320Mvar/LConn3 -- CHM7c/RConn1 -- CHM7/RConn3
  CHM7a/RConn1 -- CHM 1320Mvar/LConn1 -- CHM7/RConn1
